simulink model "vander3d"  (R2020b)
settings: Solver=ode1  StartTime=0.0  StopTime=500  FixedStep=0.002  RelTol=1e-3
values from neighbouring files (symbols this model uses):
  beta3d = 0.9    [simulate_hover.m]
  cycleGain = 0.5    [advanced_model_setup.m]    (also in setup_physical.m = 1; simulate_hover.m = 0.2)
  epsilon3d = evalin('base', 'epsilon3d')    [gainScheduling.m]    (also in simulate_hover.m = 1)
  k3d = evalin('base', 'k3d')    [gainScheduling.m]    (also in simulate_hover.m = 1.65)
settings Model: Creator=Jacob  LastModifiedBy=256444
settings DataIOCC: ReturnWorkspaceOutputs=off
settings DebuggingCC: UnconnectedInputMsg=none  UnconnectedOutputMsg=none  UnconnectedLineMsg=none
settings ModelReferenceCC: EnableRefExpFcnMdlSchedulingChecks=off

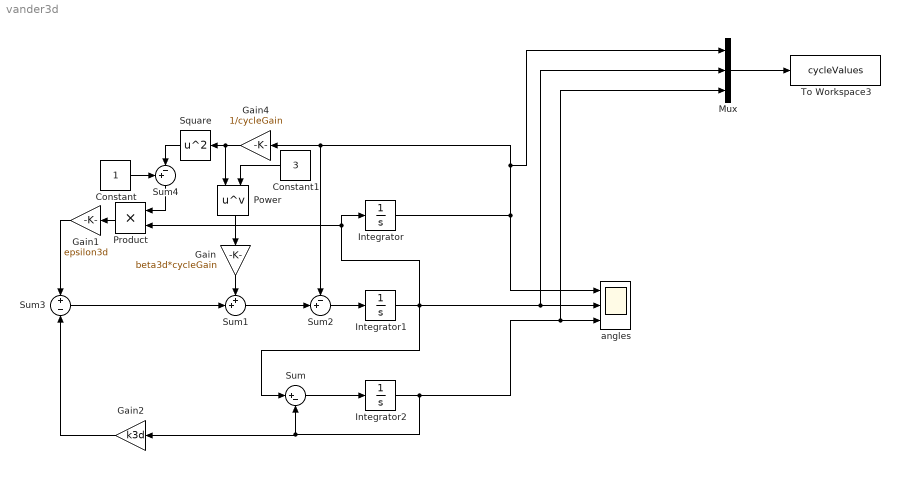
== system vander3d ==
  Constant : Constant
  Constant1 : Constant  Value=3
  Gain : Gain  Gain=beta3d*cycleGain
  Gain1 : Gain  Gain=epsilon3d
  Gain2 : Gain  Gain=k3d
  Gain4 : Gain  Gain=1/cycleGain
  Integrator : Integrator  InitialCondition=0.0001
  Integrator1 : Integrator  InitialCondition=0.0001
  Integrator2 : Integrator  InitialCondition=0.0001
  Mux : Mux  Inputs=3
  Power : Math  Operator=pow  SaturateOnIntegerOverflow=on
  Product : Product
  Square : Math  Operator=square  SaturateOnIntegerOverflow=on
  Sum : Sum  Inputs=|+-
  Sum1 : Sum  Inputs=++|
  Sum2 : Sum  Inputs=-+|
  Sum3 : Sum  Inputs=+|-
  Sum4 : Sum  Inputs=+-|
  To Workspace3 : ToWorkspace  VariableName=cycleValues  SampleTime=-1
  angles : Scope  NumInputPorts=3
  wires:
  Integrator1/1 -> Sum/1, Mux/2, angles/2, Product/2, Integrator/1
  Sum/1 -> Integrator2/1
  Integrator2/1 -> Mux/3, angles/3, Sum/2, Gain2/1
  Sum1/1 -> Sum2/2
  Sum2/1 -> Integrator1/1
  Constant1/1 -> Power/2
  Power/1 -> Gain/1
  Gain/1 -> Sum1/1
  Sum3/1 -> Sum1/2
  Sum4/1 -> Product/1
  Product/1 -> Gain1/1
  Gain1/1 -> Sum3/1
  Constant/1 -> Sum4/1
  Square/1 -> Sum4/2
  Gain2/1 -> Sum3/2
  Integrator/1 -> angles/1, Sum2/1, Gain4/1, Mux/1
  Gain4/1 -> Square/1, Power/1
  Mux/1 -> To Workspace3/1
